simulink library "inp"  (R2021b)
settings: Solver=VariableStepAuto  StartTime=0.0  StopTime=10.0  RelTol=1e-3
undefined symbols (not defined in the file): C_TASK_5MS_S, FALSE, KINP_AcoreReadyToSlp_flg_ovrdflg, KINP_AcoreReadyToSlp_flg_ovrdval, KINP_AllowMovThd_OTA_enum_ovrdflg, KINP_AllowMovThd_OTA_enum_ovrdval, KINP_APSAngleTarget_Deg_ovrdflg, KINP_APSAngleTarget_Deg_ovrdval, KINP_APSDecReq_mps2_ovrdflg, KINP_APSDecReq_mps2_ovrdval, KINP_APSDecReqA_flg_ovrdflg, KINP_APSDecReqA_flg_ovrdval, KINP_APSDFLL_cm_ovrdflg, KINP_APSDFLL_cm_ovrdval, KINP_APSDFLR_cm_ovrdflg, KINP_APSDFLR_cm_ovrdval, KINP_APSDRLL_cm_ovrdflg, KINP_APSDRLL_cm_ovrdval, KINP_APSDRLR_cm_ovrdflg, KINP_APSDRLR_cm_ovrdval, KINP_APSExitCondition_enum_ovrdflg, KINP_APSExitCondition_enum_ovrdval, KINP_APSHWVer_enum_ovrdflg, KINP_APSHWVer_enum_ovrdval, KINP_APSProgressPCT_pct_ovrdflg, KINP_APSProgressPCT_pct_ovrdval, KINP_APSPwrReq_enum_ovrdflg, KINP_APSPwrReq_enum_ovrdval, KINP_APSReq_enum_ovrdflg, KINP_APSReq_enum_ovrdval, KINP_APSRQDisplay_enum_ovrdflg, KINP_APSRQDisplay_enum_ovrdval, KINP_APSRqEPASCtrl_flg_ovrdflg, KINP_APSRqEPASCtrl_flg_ovrdval, KINP_APSShiftPosnReq_enum_ovrdval, KINP_APSShiftPosnReq_enum_ovrflg, KINP_APSSpeedCMD_kph_ovrdval, KINP_APSSpeedCMD_kph_ovrflg, KINP_APSStaSystem_enum_ovrdflg, KINP_APSStaSystem_enum_ovrdval, KINP_APSSWVer_enum_ovrdflg, KINP_APSSWVer_enum_ovrdval, KINP_APSVMCReqA_flg_ovrdval, KINP_APSVMCReqA_flg_ovrflg, KINP_APSVRqEPASCtrl_flg_ovrdflg, KINP_APSVRqEPASCtrl_flg_ovrdval, KINP_AuxBattVolmV_mV_ovrdflg, KINP_AuxBattVolmV_mV_ovrdval, KINP_CAASSta_enum_ovrdflg, KINP_CAASSta_enum_ovrdval, KINP_CAASVMCReqA_flg_ovrdval, KINP_CAASVMCReqA_flg_ovrflg, KINP_CAN1BusOff_flg_ovrdflg, KINP_CAN1BusOff_flg_ovrdval, KINP_CAN2BusOff_flg_ovrdflg, KINP_CAN2BusOff_flg_ovrdval, KINP_CAN3BusOff_flg_ovrdflg, KINP_CAN3BusOff_flg_ovrdval, KINP_CAN4BusOff_flg_ovrdflg, KINP_CAN4BusOff_flg_ovrdval ... (+152)
libraries: FVT_lib x1035, hcu_lib x1
(part 27 of 33)

== system inp/INP/CAN4/SignalCheck/ZONE_FR1 ==
  BHAL_outputs : Inport
  inp_CanValid_bus : Inport  Port=2
  ChargeInletLockSta : FVT_lib/inp/can_signal_template  SystemSampleTime=-1  VariantActivationTime=update diagram  Latency=0  AutoFrameSizeCalculation=off
      link override defval: Value=KINP_ChargeInletLockSta_flg_defval
      link override ovrdflg: Value=KINP_ChargeInletLockSta_flg_ovrdflg
      link override ovrdval: Value=KINP_ChargeInletLockSta_flg_ovrdval
  CompProEN : FVT_lib/inp/can_signal_template  SystemSampleTime=-1  VariantActivationTime=update diagram  Latency=0  AutoFrameSizeCalculation=off
      link override defval: Value=KINP_CompProEN_flg_defval
      link override ovrdflg: Value=KINP_CompProEN_flg_ovrdflg
      link override ovrdval: Value=KINP_CompProEN_flg_ovrdval
  FLTurnLPErr : FVT_lib/inp/can_signal_template  SystemSampleTime=-1  VariantActivationTime=update diagram  Latency=0  AutoFrameSizeCalculation=off
      link override defval: Value=KINP_FLTurnLPErr_flg_defval
      link override ovrdflg: Value=KINP_FLTurnLPErr_flg_ovrdflg
      link override ovrdval: Value=KINP_FLTurnLPErr_flg_ovrdval
  FLTurnLampC : FVT_lib/inp/can_signal_template  SystemSampleTime=-1  VariantActivationTime=update diagram  Latency=0  AutoFrameSizeCalculation=off
      link override defval: Value=KINP_FLTurnLampC_mA_defval
      link override ovrdflg: Value=KINP_FLTurnLampC_mA_ovrdflg
      link override ovrdval: Value=KINP_FLTurnLampC_mA_ovrdval
  FLTurnLightWarning : FVT_lib/inp/can_signal_template  SystemSampleTime=-1  VariantActivationTime=update diagram  Latency=0  AutoFrameSizeCalculation=off
      link override defval: Value=KINP_FLTurnLightWarning_flg_defval
      link override ovrdflg: Value=KINP_FLTurnLightWarning_flg_ovrdflg
      link override ovrdval: Value=KINP_FLTurnLightWarning_flg_ovrdval
  FRTurnLPErr : FVT_lib/inp/can_signal_template  SystemSampleTime=-1  VariantActivationTime=update diagram  Latency=0  AutoFrameSizeCalculation=off
      link override defval: Value=KINP_FRTurnLPErr_flg_defval
      link override ovrdflg: Value=KINP_FRTurnLPErr_flg_ovrdflg
      link override ovrdval: Value=KINP_FRTurnLPErr_flg_ovrdval
  FRTurnLampC : FVT_lib/inp/can_signal_template  SystemSampleTime=-1  VariantActivationTime=update diagram  Latency=0  AutoFrameSizeCalculation=off
      link override defval: Value=KINP_FRTurnLampC_mA_defval
      link override ovrdflg: Value=KINP_FRTurnLampC_mA_ovrdflg
      link override ovrdval: Value=KINP_FRTurnLampC_mA_ovrdval
  FRTurnLightWarning : FVT_lib/inp/can_signal_template  SystemSampleTime=-1  VariantActivationTime=update diagram  Latency=0  AutoFrameSizeCalculation=off
      link override defval: Value=KINP_FRTurnLightWarning_flg_defval
      link override ovrdflg: Value=KINP_FRTurnLightWarning_flg_ovrdflg
      link override ovrdval: Value=KINP_FRTurnLightWarning_flg_ovrdval
  FWiperAS : FVT_lib/inp/can_signal_template  SystemSampleTime=-1  VariantActivationTime=update diagram  Latency=0  AutoFrameSizeCalculation=off
      link override defval: Value=KINP_FWiperAS_flg_defval
      link override ovrdflg: Value=KINP_FWiperAS_flg_ovrdflg
      link override ovrdval: Value=KINP_FWiperAS_flg_ovrdval
  FWiperProtection : FVT_lib/inp/can_signal_template  SystemSampleTime=-1  VariantActivationTime=update diagram  Latency=0  AutoFrameSizeCalculation=off
      link override defval: Value=KINP_FWiperProtection_flg_defval
      link override ovrdflg: Value=KINP_FWiperProtection_flg_ovrdflg
      link override ovrdval: Value=KINP_FWiperProtection_flg_ovrdval
  LADBHibeamIndication : FVT_lib/inp/can_signal_template  SystemSampleTime=-1  VariantActivationTime=update diagram  Latency=0  AutoFrameSizeCalculation=off
      link override defval: Value=KINP_LADBHibeamIndication_flg_defval
      link override ovrdflg: Value=KINP_LADBHibeamIndication_flg_ovrdflg
      link override ovrdval: Value=KINP_LADBHibeamIndication_flg_ovrdval
  LADBOperationStatus : FVT_lib/inp/can_signal_template  SystemSampleTime=-1  VariantActivationTime=update diagram  Latency=0  AutoFrameSizeCalculation=off
      link override defval: Value=KINP_LADBOperationStatus_flg_defval
      link override ovrdflg: Value=KINP_LADBOperationStatus_flg_ovrdflg
      link override ovrdval: Value=KINP_LADBOperationStatus_flg_ovrdval
  LADBWarning : FVT_lib/inp/can_signal_template  SystemSampleTime=-1  VariantActivationTime=update diagram  Latency=0  AutoFrameSizeCalculation=off
      link override defval: Value=KINP_LADBWarning_flg_defval
      link override ovrdflg: Value=KINP_LADBWarning_flg_ovrdflg
      link override ovrdval: Value=KINP_LADBWarning_flg_ovrdval
  LAHBWarning : FVT_lib/inp/can_signal_template  SystemSampleTime=-1  VariantActivationTime=update diagram  Latency=0  AutoFrameSizeCalculation=off
      link override defval: Value=KINP_LAHBWarning_flg_defval
      link override ovrdflg: Value=KINP_LAHBWarning_flg_ovrdflg
      link override ovrdval: Value=KINP_LAHBWarning_flg_ovrdval
  LDRLWarning : FVT_lib/inp/can_signal_template  SystemSampleTime=-1  VariantActivationTime=update diagram  Latency=0  AutoFrameSizeCalculation=off
      link override defval: Value=KINP_LDRLWarning_flg_defval
      link override ovrdflg: Value=KINP_LDRLWarning_flg_ovrdflg
      link override ovrdval: Value=KINP_LDRLWarning_flg_ovrdval
  LLBWarning : FVT_lib/inp/can_signal_template  SystemSampleTime=-1  VariantActivationTime=update diagram  Latency=0  AutoFrameSizeCalculation=off
      link override defval: Value=KINP_LLBWarning_flg_defval
      link override ovrdflg: Value=KINP_LLBWarning_flg_ovrdflg
      link override ovrdval: Value=KINP_LLBWarning_flg_ovrdval
  LpositionLampWarning : FVT_lib/inp/can_signal_template  SystemSampleTime=-1  VariantActivationTime=update diagram  Latency=0  AutoFrameSizeCalculation=off
      link override defval: Value=KINP_LpositionLampWarning_flg_defval
      link override ovrdflg: Value=KINP_LpositionLampWarning_flg_ovrdflg
      link override ovrdval: Value=KINP_LpositionLampWarning_flg_ovrdval
  RADBHibeamIndication : FVT_lib/inp/can_signal_template  SystemSampleTime=-1  VariantActivationTime=update diagram  Latency=0  AutoFrameSizeCalculation=off
      link override defval: Value=KINP_RADBHibeamIndication_flg_defval
      link override ovrdflg: Value=KINP_RADBHibeamIndication_flg_ovrdflg
      link override ovrdval: Value=KINP_RADBHibeamIndication_flg_ovrdval
  RADBOperationStatus : FVT_lib/inp/can_signal_template  SystemSampleTime=-1  VariantActivationTime=update diagram  Latency=0  AutoFrameSizeCalculation=off
      link override defval: Value=KINP_RADBOperationStatus_flg_defval
      link override ovrdflg: Value=KINP_RADBOperationStatus_flg_ovrdflg
      link override ovrdval: Value=KINP_RADBOperationStatus_flg_ovrdval
  RADBWarning : FVT_lib/inp/can_signal_template  SystemSampleTime=-1  VariantActivationTime=update diagram  Latency=0  AutoFrameSizeCalculation=off
      link override defval: Value=KINP_RADBWarning_flg_defval
      link override ovrdflg: Value=KINP_RADBWarning_flg_ovrdflg
      link override ovrdval: Value=KINP_RADBWarning_flg_ovrdval
  RAHBWarning : FVT_lib/inp/can_signal_template  SystemSampleTime=-1  VariantActivationTime=update diagram  Latency=0  AutoFrameSizeCalculation=off
      link override defval: Value=KINP_RAHBWarning_flg_defval
      link override ovrdflg: Value=KINP_RAHBWarning_flg_ovrdflg
      link override ovrdval: Value=KINP_RAHBWarning_flg_ovrdval
  RDRLWarning : FVT_lib/inp/can_signal_template  SystemSampleTime=-1  VariantActivationTime=update diagram  Latency=0  AutoFrameSizeCalculation=off
      link override defval: Value=KINP_RDRLWarning_flg_defval
      link override ovrdflg: Value=KINP_RDRLWarning_flg_ovrdflg
      link override ovrdval: Value=KINP_RDRLWarning_flg_ovrdval
  RLBWarning : FVT_lib/inp/can_signal_template  SystemSampleTime=-1  VariantActivationTime=update diagram  Latency=0  AutoFrameSizeCalculation=off
      link override defval: Value=KINP_RLBWarning_flg_defval
      link override ovrdflg: Value=KINP_RLBWarning_flg_ovrdflg
      link override ovrdval: Value=KINP_RLBWarning_flg_ovrdval
  RpositionLampWarning : FVT_lib/inp/can_signal_template  SystemSampleTime=-1  VariantActivationTime=update diagram  Latency=0  AutoFrameSizeCalculation=off
      link override defval: Value=KINP_RpositionLampWarning_flg_defval
      link override ovrdflg: Value=KINP_RpositionLampWarning_flg_ovrdflg
      link override ovrdval: Value=KINP_RpositionLampWarning_flg_ovrdval
  Terminator_{1..33} (33 alike) : Terminator
  TrailerCheck : FVT_lib/inp/can_signal_template  SystemSampleTime=-1  VariantActivationTime=update diagram  Latency=0  AutoFrameSizeCalculation=off
      link override defval: Value=KINP_TrailerCheck_flg_defval
      link override ovrdflg: Value=KINP_TrailerCheck_flg_ovrdflg
      link override ovrdval: Value=KINP_TrailerCheck_flg_ovrdval
  TrailerModeSta : FVT_lib/inp/can_signal_template  SystemSampleTime=-1  VariantActivationTime=update diagram  Latency=0  AutoFrameSizeCalculation=off
      link override defval: Value=KINP_TrailerModeSta_enum_defval
      link override ovrdflg: Value=KINP_TrailerModeSta_enum_ovrdflg
      link override ovrdval: Value=KINP_TrailerModeSta_enum_ovrdval
  True_VHAL_ChargeInletLockSta_flg : Constant  Value=TRUE  OutDataTypeStr=boolean
  True_VHAL_CompProEN_flg : Constant  Value=TRUE  OutDataTypeStr=boolean
  True_VHAL_FLTurnLPErr_flg : Constant  Value=TRUE  OutDataTypeStr=boolean
  True_VHAL_FLTurnLampC_mA : Constant  Value=TRUE  OutDataTypeStr=boolean
  True_VHAL_FLTurnLightWarning_flg : Constant  Value=TRUE  OutDataTypeStr=boolean
  True_VHAL_FRTurnLPErr_flg : Constant  Value=TRUE  OutDataTypeStr=boolean
  True_VHAL_FRTurnLampC_mA : Constant  Value=TRUE  OutDataTypeStr=boolean
  True_VHAL_FRTurnLightWarning_flg : Constant  Value=TRUE  OutDataTypeStr=boolean
  True_VHAL_FWiperAS_flg : Constant  Value=TRUE  OutDataTypeStr=boolean
  True_VHAL_FWiperProtection_flg : Constant  Value=TRUE  OutDataTypeStr=boolean
  True_VHAL_LADBHibeamIndication_flg : Constant  Value=TRUE  OutDataTypeStr=boolean
  True_VHAL_LADBOperationStatus_flg : Constant  Value=TRUE  OutDataTypeStr=boolean
  True_VHAL_LADBWarning_flg : Constant  Value=TRUE  OutDataTypeStr=boolean
  True_VHAL_LAHBWarning_flg : Constant  Value=TRUE  OutDataTypeStr=boolean
  True_VHAL_LDRLWarning_flg : Constant  Value=TRUE  OutDataTypeStr=boolean
  True_VHAL_LLBWarning_flg : Constant  Value=TRUE  OutDataTypeStr=boolean
  True_VHAL_LpositionLampWarning_flg : Constant  Value=TRUE  OutDataTypeStr=boolean
  True_VHAL_RADBHibeamIndication_flg : Constant  Value=TRUE  OutDataTypeStr=boolean
  True_VHAL_RADBOperationStatus_flg : Constant  Value=TRUE  OutDataTypeStr=boolean
  True_VHAL_RADBWarning_flg : Constant  Value=TRUE  OutDataTypeStr=boolean
  True_VHAL_RAHBWarning_flg : Constant  Value=TRUE  OutDataTypeStr=boolean
  True_VHAL_RDRLWarning_flg : Constant  Value=TRUE  OutDataTypeStr=boolean
  True_VHAL_RLBWarning_flg : Constant  Value=TRUE  OutDataTypeStr=boolean
  True_VHAL_RpositionLampWarning_flg : Constant  Value=TRUE  OutDataTypeStr=boolean
  True_VHAL_TrailerCheck_flg : Constant  Value=TRUE  OutDataTypeStr=boolean
  True_VHAL_TrailerModeSta_enum : Constant  Value=TRUE  OutDataTypeStr=boolean
  True_VHAL_ZFRBCMChargerDoorSWSta_flg : Constant  Value=TRUE  OutDataTypeStr=boolean
  True_VHAL_ZFRBCMHRLTurnLPNormalSta_flg : Constant  Value=TRUE  OutDataTypeStr=boolean
  True_VHAL_ZFRBCMHRRTurnLPHNormalSta_flg : Constant  Value=TRUE  OutDataTypeStr=boolean
  True_VHAL_ZFRTHCMCLEVentActYSta_pct : Constant  Value=TRUE  OutDataTypeStr=boolean
  True_VHAL_ZFRTHCMCREVentActYSta_pct : Constant  Value=TRUE  OutDataTypeStr=boolean
  True_VHAL_ZFRTHCMDrEVentActYSta_pct : Constant  Value=TRUE  OutDataTypeStr=boolean
  True_VHAL_ZFRTHCMPsEVentActYSta_pct : Constant  Value=TRUE  OutDataTypeStr=boolean
  ZFRBCMChargerDoorSWSta : FVT_lib/inp/can_signal_template  SystemSampleTime=-1  VariantActivationTime=update diagram  Latency=0  AutoFrameSizeCalculation=off
      link override defval: Value=KINP_ZFRBCMChargerDoorSWSta_flg_defval
      link override ovrdflg: Value=KINP_ZFRBCMChargerDoorSWSta_flg_ovrdflg
      link override ovrdval: Value=KINP_ZFRBCMChargerDoorSWSta_flg_ovrdval
  ZFRBCMHRLTurnLPNormalSta : FVT_lib/inp/can_signal_template  SystemSampleTime=-1  VariantActivationTime=update diagram  Latency=0  AutoFrameSizeCalculation=off
      link override defval: Value=KINP_ZFRBCMHRLTurnLPNormalSta_flg_defval
      link override ovrdflg: Value=KINP_ZFRBCMHRLTurnLPNormalSta_flg_ovrdflg
      link override ovrdval: Value=KINP_ZFRBCMHRLTurnLPNormalSta_flg_ovrdval
  ZFRBCMHRRTurnLPHNormalSta : FVT_lib/inp/can_signal_template  SystemSampleTime=-1  VariantActivationTime=update diagram  Latency=0  AutoFrameSizeCalculation=off
      link override defval: Value=KINP_ZFRBCMHRRTurnLPHNormalSta_flg_defval
      link override ovrdflg: Value=KINP_ZFRBCMHRRTurnLPHNormalSta_flg_ovrdflg
      link override ovrdval: Value=KINP_ZFRBCMHRRTurnLPHNormalSta_flg_ovrdval
  ZFRTHCMCLEVentActYSta : FVT_lib/inp/can_signal_template  SystemSampleTime=-1  VariantActivationTime=update diagram  Latency=0  AutoFrameSizeCalculation=off
      link override defval: Value=KINP_ZFRTHCMCLEVentActYSta_pct_defval
      link override ovrdflg: Value=KINP_ZFRTHCMCLEVentActYSta_pct_ovrdflg
      link override ovrdval: Value=KINP_ZFRTHCMCLEVentActYSta_pct_ovrdval
  ZFRTHCMCREVentActYSta : FVT_lib/inp/can_signal_template  SystemSampleTime=-1  VariantActivationTime=update diagram  Latency=0  AutoFrameSizeCalculation=off
      link override defval: Value=KINP_ZFRTHCMCREVentActYSta_pct_defval
      link override ovrdflg: Value=KINP_ZFRTHCMCREVentActYSta_pct_ovrdflg
      link override ovrdval: Value=KINP_ZFRTHCMCREVentActYSta_pct_ovrdval
  ZFRTHCMDrEVentActYSta : FVT_lib/inp/can_signal_template  SystemSampleTime=-1  VariantActivationTime=update diagram  Latency=0  AutoFrameSizeCalculation=off
      link override defval: Value=KINP_ZFRTHCMDrEVentActYSta_pct_defval
      link override ovrdflg: Value=KINP_ZFRTHCMDrEVentActYSta_pct_ovrdflg
      link override ovrdval: Value=KINP_ZFRTHCMDrEVentActYSta_pct_ovrdval
  ZFRTHCMPsEVentActYSta : FVT_lib/inp/can_signal_template  SystemSampleTime=-1  VariantActivationTime=update diagram  Latency=0  AutoFrameSizeCalculation=off
      link override defval: Value=KINP_ZFRTHCMPsEVentActYSta_pct_defval
      link override ovrdflg: Value=KINP_ZFRTHCMPsEVentActYSta_pct_ovrdflg
      link override ovrdval: Value=KINP_ZFRTHCMPsEVentActYSta_pct_ovrdval
  slr1_{1..33} (33 alike) : BusSelector  OutputSignals=VINP_CANMsgValidZONEFR1_flg
  slr_VHAL_ChargeInletLockSta_flg : BusSelector  OutputSignals=VHAL_ChargeInletLockSta_flg
  slr_VHAL_CompProEN_flg : BusSelector  OutputSignals=VHAL_CompProEN_flg
  slr_VHAL_FLTurnLPErr_flg : BusSelector  OutputSignals=VHAL_FLTurnLPErr_flg
  slr_VHAL_FLTurnLampC_mA : BusSelector  OutputSignals=VHAL_FLTurnLampC_mA
  slr_VHAL_FLTurnLightWarning_flg : BusSelector  OutputSignals=VHAL_FLTurnLightWarning_flg
  slr_VHAL_FRTurnLPErr_flg : BusSelector  OutputSignals=VHAL_FRTurnLPErr_flg
  slr_VHAL_FRTurnLampC_mA : BusSelector  OutputSignals=VHAL_FRTurnLampC_mA
  slr_VHAL_FRTurnLightWarning_flg : BusSelector  OutputSignals=VHAL_FRTurnLightWarning_flg
  slr_VHAL_FWiperAS_flg : BusSelector  OutputSignals=VHAL_FWiperAS_flg
  slr_VHAL_FWiperProtection_flg : BusSelector  OutputSignals=VHAL_FWiperProtection_flg
  slr_VHAL_LADBHibeamIndication_flg : BusSelector  OutputSignals=VHAL_LADBHibeamIndication_flg
  slr_VHAL_LADBOperationStatus_flg : BusSelector  OutputSignals=VHAL_LADBOperationStatus_flg
  slr_VHAL_LADBWarning_flg : BusSelector  OutputSignals=VHAL_LADBWarning_flg
  slr_VHAL_LAHBWarning_flg : BusSelector  OutputSignals=VHAL_LAHBWarning_flg
  slr_VHAL_LDRLWarning_flg : BusSelector  OutputSignals=VHAL_LDRLWarning_flg
  slr_VHAL_LLBWarning_flg : BusSelector  OutputSignals=VHAL_LLBWarning_flg
  slr_VHAL_LpositionLampWarning_flg : BusSelector  OutputSignals=VHAL_LpositionLampWarning_flg
  slr_VHAL_RADBHibeamIndication_flg : BusSelector  OutputSignals=VHAL_RADBHibeamIndication_flg
  slr_VHAL_RADBOperationStatus_flg : BusSelector  OutputSignals=VHAL_RADBOperationStatus_flg
  slr_VHAL_RADBWarning_flg : BusSelector  OutputSignals=VHAL_RADBWarning_flg
  slr_VHAL_RAHBWarning_flg : BusSelector  OutputSignals=VHAL_RAHBWarning_flg
  slr_VHAL_RDRLWarning_flg : BusSelector  OutputSignals=VHAL_RDRLWarning_flg
  slr_VHAL_RLBWarning_flg : BusSelector  OutputSignals=VHAL_RLBWarning_flg
  slr_VHAL_RpositionLampWarning_flg : BusSelector  OutputSignals=VHAL_RpositionLampWarning_flg
  slr_VHAL_TrailerCheck_flg : BusSelector  OutputSignals=VHAL_TrailerCheck_flg
  slr_VHAL_TrailerModeSta_enum : BusSelector  OutputSignals=VHAL_TrailerModeSta_enum
  slr_VHAL_ZFRBCMChargerDoorSWSta_flg : BusSelector  OutputSignals=VHAL_ZFRBCMChargerDoorSWSta_flg
  slr_VHAL_ZFRBCMHRLTurnLPNormalSta_flg : BusSelector  OutputSignals=VHAL_ZFRBCMHRLTurnLPNormalSta_flg
  slr_VHAL_ZFRBCMHRRTurnLPHNormalSta_flg : BusSelector  OutputSignals=VHAL_ZFRBCMHRRTurnLPHNormalSta_flg
  slr_VHAL_ZFRTHCMCLEVentActYSta_pct : BusSelector  OutputSignals=VHAL_ZFRTHCMCLEVentActYSta_pct
  slr_VHAL_ZFRTHCMCREVentActYSta_pct : BusSelector  OutputSignals=VHAL_ZFRTHCMCREVentActYSta_pct
  slr_VHAL_ZFRTHCMDrEVentActYSta_pct : BusSelector  OutputSignals=VHAL_ZFRTHCMDrEVentActYSta_pct
  slr_VHAL_ZFRTHCMPsEVentActYSta_pct : BusSelector  OutputSignals=VHAL_ZFRTHCMPsEVentActYSta_pct
  VINP_ChargeInletLockSta_flg : Outport
  VINP_CompProEN_flg : Outport  Port=2
  VINP_FLTurnLPErr_flg : Outport  Port=3
  VINP_FLTurnLampC_mA : Outport  Port=4
  VINP_FLTurnLightWarning_flg : Outport  Port=5
  VINP_FRTurnLPErr_flg : Outport  Port=6
  VINP_FRTurnLampC_mA : Outport  Port=7
  VINP_FRTurnLightWarning_flg : Outport  Port=8
  VINP_FWiperAS_flg : Outport  Port=9
  VINP_FWiperProtection_flg : Outport  Port=10
  VINP_LADBHibeamIndication_flg : Outport  Port=11
  VINP_LADBOperationStatus_flg : Outport  Port=12
  VINP_LADBWarning_flg : Outport  Port=13
  VINP_LAHBWarning_flg : Outport  Port=14
  VINP_LDRLWarning_flg : Outport  Port=15
  VINP_LLBWarning_flg : Outport  Port=16
  VINP_LpositionLampWarning_flg : Outport  Port=17
  VINP_RADBHibeamIndication_flg : Outport  Port=18
  VINP_RADBOperationStatus_flg : Outport  Port=19
  VINP_RADBWarning_flg : Outport  Port=20
  VINP_RAHBWarning_flg : Outport  Port=21
  VINP_RDRLWarning_flg : Outport  Port=22
  VINP_RLBWarning_flg : Outport  Port=23
  VINP_RpositionLampWarning_flg : Outport  Port=24
  VINP_TrailerCheck_flg : Outport  Port=25
  VINP_TrailerModeSta_enum : Outport  Port=26
  VINP_ZFRBCMChargerDoorSWSta_flg : Outport  Port=27
  VINP_ZFRBCMHRLTurnLPNormalSta_flg : Outport  Port=28
  VINP_ZFRBCMHRRTurnLPHNormalSta_flg : Outport  Port=29
  VINP_ZFRTHCMCLEVentActYSta_pct : Outport  Port=30
  VINP_ZFRTHCMCREVentActYSta_pct : Outport  Port=31
  VINP_ZFRTHCMDrEVentActYSta_pct : Outport  Port=32
  VINP_ZFRTHCMPsEVentActYSta_pct : Outport  Port=33
  wires:
  BHAL_outputs/1 -> [BHAL_outputs]
  inp_CanValid_bus/1 -> [inp_CanValid_bus]
  [BHAL_outputs] -> slr_VHAL_ChargeInletLockSta_flg/1
  slr_VHAL_ChargeInletLockSta_flg/1 -> ChargeInletLockSta/1  "<VHAL_ChargeInletLockSta_flg>"
  True_VHAL_ChargeInletLockSta_flg/1 -> ChargeInletLockSta/2
  [inp_CanValid_bus] -> slr1_1/1
  slr1_1/1 -> ChargeInletLockSta/3  "<VINP_CANMsgValidZONEFR1_flg>"
  ChargeInletLockSta/1 -> VINP_ChargeInletLockSta_flg/1  "VINP_ChargeInletLockSta_flg"
  ChargeInletLockSta/2 -> Terminator_1/1
  [BHAL_outputs] -> slr_VHAL_CompProEN_flg/1
  slr_VHAL_CompProEN_flg/1 -> CompProEN/1  "<VHAL_CompProEN_flg>"
  True_VHAL_CompProEN_flg/1 -> CompProEN/2
  [inp_CanValid_bus] -> slr1_2/1
  slr1_2/1 -> CompProEN/3  "<VINP_CANMsgValidZONEFR1_flg>"
  CompProEN/1 -> VINP_CompProEN_flg/1  "VINP_CompProEN_flg"
  CompProEN/2 -> Terminator_2/1
  [BHAL_outputs] -> slr_VHAL_FLTurnLPErr_flg/1
  slr_VHAL_FLTurnLPErr_flg/1 -> FLTurnLPErr/1  "<VHAL_FLTurnLPErr_flg>"
  True_VHAL_FLTurnLPErr_flg/1 -> FLTurnLPErr/2
  [inp_CanValid_bus] -> slr1_3/1
  slr1_3/1 -> FLTurnLPErr/3  "<VINP_CANMsgValidZONEFR1_flg>"
  FLTurnLPErr/1 -> VINP_FLTurnLPErr_flg/1  "VINP_FLTurnLPErr_flg"
  FLTurnLPErr/2 -> Terminator_3/1
  [BHAL_outputs] -> slr_VHAL_FLTurnLampC_mA/1
  slr_VHAL_FLTurnLampC_mA/1 -> FLTurnLampC/1  "<VHAL_FLTurnLampC_mA>"
  True_VHAL_FLTurnLampC_mA/1 -> FLTurnLampC/2
  [inp_CanValid_bus] -> slr1_4/1
  slr1_4/1 -> FLTurnLampC/3  "<VINP_CANMsgValidZONEFR1_flg>"
  FLTurnLampC/1 -> VINP_FLTurnLampC_mA/1  "VINP_FLTurnLampC_mA"
  FLTurnLampC/2 -> Terminator_4/1
  [BHAL_outputs] -> slr_VHAL_FLTurnLightWarning_flg/1
  slr_VHAL_FLTurnLightWarning_flg/1 -> FLTurnLightWarning/1  "<VHAL_FLTurnLightWarning_flg>"
  True_VHAL_FLTurnLightWarning_flg/1 -> FLTurnLightWarning/2
  [inp_CanValid_bus] -> slr1_5/1
  slr1_5/1 -> FLTurnLightWarning/3  "<VINP_CANMsgValidZONEFR1_flg>"
  FLTurnLightWarning/1 -> VINP_FLTurnLightWarning_flg/1  "VINP_FLTurnLightWarning_flg"
  FLTurnLightWarning/2 -> Terminator_5/1
  [BHAL_outputs] -> slr_VHAL_FRTurnLPErr_flg/1
  slr_VHAL_FRTurnLPErr_flg/1 -> FRTurnLPErr/1  "<VHAL_FRTurnLPErr_flg>"
  True_VHAL_FRTurnLPErr_flg/1 -> FRTurnLPErr/2
  [inp_CanValid_bus] -> slr1_6/1
  slr1_6/1 -> FRTurnLPErr/3  "<VINP_CANMsgValidZONEFR1_flg>"
  FRTurnLPErr/1 -> VINP_FRTurnLPErr_flg/1  "VINP_FRTurnLPErr_flg"
  FRTurnLPErr/2 -> Terminator_6/1
  [BHAL_outputs] -> slr_VHAL_FRTurnLampC_mA/1
  slr_VHAL_FRTurnLampC_mA/1 -> FRTurnLampC/1  "<VHAL_FRTurnLampC_mA>"
  True_VHAL_FRTurnLampC_mA/1 -> FRTurnLampC/2
  [inp_CanValid_bus] -> slr1_7/1
  slr1_7/1 -> FRTurnLampC/3  "<VINP_CANMsgValidZONEFR1_flg>"
  FRTurnLampC/1 -> VINP_FRTurnLampC_mA/1  "VINP_FRTurnLampC_mA"
  FRTurnLampC/2 -> Terminator_7/1
  [BHAL_outputs] -> slr_VHAL_FRTurnLightWarning_flg/1
  slr_VHAL_FRTurnLightWarning_flg/1 -> FRTurnLightWarning/1  "<VHAL_FRTurnLightWarning_flg>"
  True_VHAL_FRTurnLightWarning_flg/1 -> FRTurnLightWarning/2
  [inp_CanValid_bus] -> slr1_8/1
  slr1_8/1 -> FRTurnLightWarning/3  "<VINP_CANMsgValidZONEFR1_flg>"
  FRTurnLightWarning/1 -> VINP_FRTurnLightWarning_flg/1  "VINP_FRTurnLightWarning_flg"
  FRTurnLightWarning/2 -> Terminator_8/1
  [BHAL_outputs] -> slr_VHAL_FWiperAS_flg/1
  slr_VHAL_FWiperAS_flg/1 -> FWiperAS/1  "<VHAL_FWiperAS_flg>"
  True_VHAL_FWiperAS_flg/1 -> FWiperAS/2
  [inp_CanValid_bus] -> slr1_9/1
  slr1_9/1 -> FWiperAS/3  "<VINP_CANMsgValidZONEFR1_flg>"
  FWiperAS/1 -> VINP_FWiperAS_flg/1  "VINP_FWiperAS_flg"
  FWiperAS/2 -> Terminator_9/1
  [BHAL_outputs] -> slr_VHAL_FWiperProtection_flg/1
  slr_VHAL_FWiperProtection_flg/1 -> FWiperProtection/1  "<VHAL_FWiperProtection_flg>"
  True_VHAL_FWiperProtection_flg/1 -> FWiperProtection/2
  [inp_CanValid_bus] -> slr1_10/1
  slr1_10/1 -> FWiperProtection/3  "<VINP_CANMsgValidZONEFR1_flg>"
  FWiperProtection/1 -> VINP_FWiperProtection_flg/1  "VINP_FWiperProtection_flg"
  FWiperProtection/2 -> Terminator_10/1
  [BHAL_outputs] -> slr_VHAL_LADBHibeamIndication_flg/1
  slr_VHAL_LADBHibeamIndication_flg/1 -> LADBHibeamIndication/1  "<VHAL_LADBHibeamIndication_flg>"
  True_VHAL_LADBHibeamIndication_flg/1 -> LADBHibeamIndication/2
  [inp_CanValid_bus] -> slr1_11/1
  slr1_11/1 -> LADBHibeamIndication/3  "<VINP_CANMsgValidZONEFR1_flg>"
  LADBHibeamIndication/1 -> VINP_LADBHibeamIndication_flg/1  "VINP_LADBHibeamIndication_flg"
  LADBHibeamIndication/2 -> Terminator_11/1
  [BHAL_outputs] -> slr_VHAL_LADBOperationStatus_flg/1
  slr_VHAL_LADBOperationStatus_flg/1 -> LADBOperationStatus/1  "<VHAL_LADBOperationStatus_flg>"
  True_VHAL_LADBOperationStatus_flg/1 -> LADBOperationStatus/2
  [inp_CanValid_bus] -> slr1_12/1
  slr1_12/1 -> LADBOperationStatus/3  "<VINP_CANMsgValidZONEFR1_flg>"
  LADBOperationStatus/1 -> VINP_LADBOperationStatus_flg/1  "VINP_LADBOperationStatus_flg"
  LADBOperationStatus/2 -> Terminator_12/1
  [BHAL_outputs] -> slr_VHAL_LADBWarning_flg/1
  slr_VHAL_LADBWarning_flg/1 -> LADBWarning/1  "<VHAL_LADBWarning_flg>"
  True_VHAL_LADBWarning_flg/1 -> LADBWarning/2
  [inp_CanValid_bus] -> slr1_13/1
  slr1_13/1 -> LADBWarning/3  "<VINP_CANMsgValidZONEFR1_flg>"
  LADBWarning/1 -> VINP_LADBWarning_flg/1  "VINP_LADBWarning_flg"
  LADBWarning/2 -> Terminator_13/1
  [BHAL_outputs] -> slr_VHAL_LAHBWarning_flg/1
  slr_VHAL_LAHBWarning_flg/1 -> LAHBWarning/1  "<VHAL_LAHBWarning_flg>"
  True_VHAL_LAHBWarning_flg/1 -> LAHBWarning/2
  [inp_CanValid_bus] -> slr1_14/1
  slr1_14/1 -> LAHBWarning/3  "<VINP_CANMsgValidZONEFR1_flg>"
  LAHBWarning/1 -> VINP_LAHBWarning_flg/1  "VINP_LAHBWarning_flg"
  LAHBWarning/2 -> Terminator_14/1
  [BHAL_outputs] -> slr_VHAL_LDRLWarning_flg/1
  slr_VHAL_LDRLWarning_flg/1 -> LDRLWarning/1  "<VHAL_LDRLWarning_flg>"
  True_VHAL_LDRLWarning_flg/1 -> LDRLWarning/2
  [inp_CanValid_bus] -> slr1_15/1
  slr1_15/1 -> LDRLWarning/3  "<VINP_CANMsgValidZONEFR1_flg>"
  LDRLWarning/1 -> VINP_LDRLWarning_flg/1  "VINP_LDRLWarning_flg"
  LDRLWarning/2 -> Terminator_15/1
  [BHAL_outputs] -> slr_VHAL_LLBWarning_flg/1
  slr_VHAL_LLBWarning_flg/1 -> LLBWarning/1  "<VHAL_LLBWarning_flg>"
  True_VHAL_LLBWarning_flg/1 -> LLBWarning/2
  [inp_CanValid_bus] -> slr1_16/1
  slr1_16/1 -> LLBWarning/3  "<VINP_CANMsgValidZONEFR1_flg>"
  LLBWarning/1 -> VINP_LLBWarning_flg/1  "VINP_LLBWarning_flg"
  LLBWarning/2 -> Terminator_16/1
  [BHAL_outputs] -> slr_VHAL_LpositionLampWarning_flg/1
  slr_VHAL_LpositionLampWarning_flg/1 -> LpositionLampWarning/1  "<VHAL_LpositionLampWarning_flg>"
  True_VHAL_LpositionLampWarning_flg/1 -> LpositionLampWarning/2
  [inp_CanValid_bus] -> slr1_17/1
  slr1_17/1 -> LpositionLampWarning/3  "<VINP_CANMsgValidZONEFR1_flg>"
  LpositionLampWarning/1 -> VINP_LpositionLampWarning_flg/1  "VINP_LpositionLampWarning_flg"
  LpositionLampWarning/2 -> Terminator_17/1
  [BHAL_outputs] -> slr_VHAL_RADBHibeamIndication_flg/1
  slr_VHAL_RADBHibeamIndication_flg/1 -> RADBHibeamIndication/1  "<VHAL_RADBHibeamIndication_flg>"
  True_VHAL_RADBHibeamIndication_flg/1 -> RADBHibeamIndication/2
  [inp_CanValid_bus] -> slr1_18/1
  slr1_18/1 -> RADBHibeamIndication/3  "<VINP_CANMsgValidZONEFR1_flg>"
  RADBHibeamIndication/1 -> VINP_RADBHibeamIndication_flg/1  "VINP_RADBHibeamIndication_flg"
  RADBHibeamIndication/2 -> Terminator_18/1
  [BHAL_outputs] -> slr_VHAL_RADBOperationStatus_flg/1
  slr_VHAL_RADBOperationStatus_flg/1 -> RADBOperationStatus/1  "<VHAL_RADBOperationStatus_flg>"
  True_VHAL_RADBOperationStatus_flg/1 -> RADBOperationStatus/2
  [inp_CanValid_bus] -> slr1_19/1
  slr1_19/1 -> RADBOperationStatus/3  "<VINP_CANMsgValidZONEFR1_flg>"
  RADBOperationStatus/1 -> VINP_RADBOperationStatus_flg/1  "VINP_RADBOperationStatus_flg"
  RADBOperationStatus/2 -> Terminator_19/1
  [BHAL_outputs] -> slr_VHAL_RADBWarning_flg/1
  slr_VHAL_RADBWarning_flg/1 -> RADBWarning/1  "<VHAL_RADBWarning_flg>"
  True_VHAL_RADBWarning_flg/1 -> RADBWarning/2
  [inp_CanValid_bus] -> slr1_20/1
  slr1_20/1 -> RADBWarning/3  "<VINP_CANMsgValidZONEFR1_flg>"
  RADBWarning/1 -> VINP_RADBWarning_flg/1  "VINP_RADBWarning_flg"
  RADBWarning/2 -> Terminator_20/1
  [BHAL_outputs] -> slr_VHAL_RAHBWarning_flg/1
  slr_VHAL_RAHBWarning_flg/1 -> RAHBWarning/1  "<VHAL_RAHBWarning_flg>"
  True_VHAL_RAHBWarning_flg/1 -> RAHBWarning/2
  [inp_CanValid_bus] -> slr1_21/1
  slr1_21/1 -> RAHBWarning/3  "<VINP_CANMsgValidZONEFR1_flg>"
  RAHBWarning/1 -> VINP_RAHBWarning_flg/1  "VINP_RAHBWarning_flg"
  RAHBWarning/2 -> Terminator_21/1
  [BHAL_outputs] -> slr_VHAL_RDRLWarning_flg/1
  slr_VHAL_RDRLWarning_flg/1 -> RDRLWarning/1  "<VHAL_RDRLWarning_flg>"
  True_VHAL_RDRLWarning_flg/1 -> RDRLWarning/2
  [inp_CanValid_bus] -> slr1_22/1
  slr1_22/1 -> RDRLWarning/3  "<VINP_CANMsgValidZONEFR1_flg>"
  RDRLWarning/1 -> VINP_RDRLWarning_flg/1  "VINP_RDRLWarning_flg"
  RDRLWarning/2 -> Terminator_22/1
  [BHAL_outputs] -> slr_VHAL_RLBWarning_flg/1
  slr_VHAL_RLBWarning_flg/1 -> RLBWarning/1  "<VHAL_RLBWarning_flg>"
  True_VHAL_RLBWarning_flg/1 -> RLBWarning/2
  [inp_CanValid_bus] -> slr1_23/1
  slr1_23/1 -> RLBWarning/3  "<VINP_CANMsgValidZONEFR1_flg>"
  RLBWarning/1 -> VINP_RLBWarning_flg/1  "VINP_RLBWarning_flg"
  RLBWarning/2 -> Terminator_23/1
  [BHAL_outputs] -> slr_VHAL_RpositionLampWarning_flg/1
  slr_VHAL_RpositionLampWarning_flg/1 -> RpositionLampWarning/1  "<VHAL_RpositionLampWarning_flg>"
  True_VHAL_RpositionLampWarning_flg/1 -> RpositionLampWarning/2
  [inp_CanValid_bus] -> slr1_24/1
  slr1_24/1 -> RpositionLampWarning/3  "<VINP_CANMsgValidZONEFR1_flg>"
  RpositionLampWarning/1 -> VINP_RpositionLampWarning_flg/1  "VINP_RpositionLampWarning_flg"
  RpositionLampWarning/2 -> Terminator_24/1
  [BHAL_outputs] -> slr_VHAL_TrailerCheck_flg/1
  slr_VHAL_TrailerCheck_flg/1 -> TrailerCheck/1  "<VHAL_TrailerCheck_flg>"
  True_VHAL_TrailerCheck_flg/1 -> TrailerCheck/2
  [inp_CanValid_bus] -> slr1_25/1
  slr1_25/1 -> TrailerCheck/3  "<VINP_CANMsgValidZONEFR1_flg>"
  TrailerCheck/1 -> VINP_TrailerCheck_flg/1  "VINP_TrailerCheck_flg"
  TrailerCheck/2 -> Terminator_25/1
  [BHAL_outputs] -> slr_VHAL_TrailerModeSta_enum/1
  slr_VHAL_TrailerModeSta_enum/1 -> TrailerModeSta/1  "<VHAL_TrailerModeSta_enum>"
  True_VHAL_TrailerModeSta_enum/1 -> TrailerModeSta/2
  [inp_CanValid_bus] -> slr1_26/1
  slr1_26/1 -> TrailerModeSta/3  "<VINP_CANMsgValidZONEFR1_flg>"
  TrailerModeSta/1 -> VINP_TrailerModeSta_enum/1  "VINP_TrailerModeSta_enum"
  TrailerModeSta/2 -> Terminator_26/1
  [BHAL_outputs] -> slr_VHAL_ZFRBCMChargerDoorSWSta_flg/1
  slr_VHAL_ZFRBCMChargerDoorSWSta_flg/1 -> ZFRBCMChargerDoorSWSta/1  "<VHAL_ZFRBCMChargerDoorSWSta_flg>"
  True_VHAL_ZFRBCMChargerDoorSWSta_flg/1 -> ZFRBCMChargerDoorSWSta/2
  [inp_CanValid_bus] -> slr1_27/1
  slr1_27/1 -> ZFRBCMChargerDoorSWSta/3  "<VINP_CANMsgValidZONEFR1_flg>"
  ZFRBCMChargerDoorSWSta/1 -> VINP_ZFRBCMChargerDoorSWSta_flg/1  "VINP_ZFRBCMChargerDoorSWSta_flg"
  ZFRBCMChargerDoorSWSta/2 -> Terminator_27/1
  [BHAL_outputs] -> slr_VHAL_ZFRBCMHRLTurnLPNormalSta_flg/1
  slr_VHAL_ZFRBCMHRLTurnLPNormalSta_flg/1 -> ZFRBCMHRLTurnLPNormalSta/1  "<VHAL_ZFRBCMHRLTurnLPNormalSta_flg>"
  True_VHAL_ZFRBCMHRLTurnLPNormalSta_flg/1 -> ZFRBCMHRLTurnLPNormalSta/2
  [inp_CanValid_bus] -> slr1_28/1
  slr1_28/1 -> ZFRBCMHRLTurnLPNormalSta/3  "<VINP_CANMsgValidZONEFR1_flg>"
  ZFRBCMHRLTurnLPNormalSta/1 -> VINP_ZFRBCMHRLTurnLPNormalSta_flg/1  "VINP_ZFRBCMHRLTurnLPNormalSta_flg"
  ZFRBCMHRLTurnLPNormalSta/2 -> Terminator_28/1
  [BHAL_outputs] -> slr_VHAL_ZFRBCMHRRTurnLPHNormalSta_flg/1
  slr_VHAL_ZFRBCMHRRTurnLPHNormalSta_flg/1 -> ZFRBCMHRRTurnLPHNormalSta/1  "<VHAL_ZFRBCMHRRTurnLPHNormalSta_flg>"
  True_VHAL_ZFRBCMHRRTurnLPHNormalSta_flg/1 -> ZFRBCMHRRTurnLPHNormalSta/2
  [inp_CanValid_bus] -> slr1_29/1
  slr1_29/1 -> ZFRBCMHRRTurnLPHNormalSta/3  "<VINP_CANMsgValidZONEFR1_flg>"
  ZFRBCMHRRTurnLPHNormalSta/1 -> VINP_ZFRBCMHRRTurnLPHNormalSta_flg/1  "VINP_ZFRBCMHRRTurnLPHNormalSta_flg"
  ZFRBCMHRRTurnLPHNormalSta/2 -> Terminator_29/1
  [BHAL_outputs] -> slr_VHAL_ZFRTHCMCLEVentActYSta_pct/1
  slr_VHAL_ZFRTHCMCLEVentActYSta_pct/1 -> ZFRTHCMCLEVentActYSta/1  "<VHAL_ZFRTHCMCLEVentActYSta_pct>"
  True_VHAL_ZFRTHCMCLEVentActYSta_pct/1 -> ZFRTHCMCLEVentActYSta/2
  [inp_CanValid_bus] -> slr1_30/1
  slr1_30/1 -> ZFRTHCMCLEVentActYSta/3  "<VINP_CANMsgValidZONEFR1_flg>"
  ZFRTHCMCLEVentActYSta/1 -> VINP_ZFRTHCMCLEVentActYSta_pct/1  "VINP_ZFRTHCMCLEVentActYSta_pct"
  ZFRTHCMCLEVentActYSta/2 -> Terminator_30/1
  [BHAL_outputs] -> slr_VHAL_ZFRTHCMCREVentActYSta_pct/1
  slr_VHAL_ZFRTHCMCREVentActYSta_pct/1 -> ZFRTHCMCREVentActYSta/1  "<VHAL_ZFRTHCMCREVentActYSta_pct>"
  True_VHAL_ZFRTHCMCREVentActYSta_pct/1 -> ZFRTHCMCREVentActYSta/2
  [inp_CanValid_bus] -> slr1_31/1
  slr1_31/1 -> ZFRTHCMCREVentActYSta/3  "<VINP_CANMsgValidZONEFR1_flg>"
  ZFRTHCMCREVentActYSta/1 -> VINP_ZFRTHCMCREVentActYSta_pct/1  "VINP_ZFRTHCMCREVentActYSta_pct"
  ZFRTHCMCREVentActYSta/2 -> Terminator_31/1
  [BHAL_outputs] -> slr_VHAL_ZFRTHCMDrEVentActYSta_pct/1
  slr_VHAL_ZFRTHCMDrEVentActYSta_pct/1 -> ZFRTHCMDrEVentActYSta/1  "<VHAL_ZFRTHCMDrEVentActYSta_pct>"
  True_VHAL_ZFRTHCMDrEVentActYSta_pct/1 -> ZFRTHCMDrEVentActYSta/2
  [inp_CanValid_bus] -> slr1_32/1
  slr1_32/1 -> ZFRTHCMDrEVentActYSta/3  "<VINP_CANMsgValidZONEFR1_flg>"
  ZFRTHCMDrEVentActYSta/1 -> VINP_ZFRTHCMDrEVentActYSta_pct/1  "VINP_ZFRTHCMDrEVentActYSta_pct"
  ZFRTHCMDrEVentActYSta/2 -> Terminator_32/1
  [BHAL_outputs] -> slr_VHAL_ZFRTHCMPsEVentActYSta_pct/1
  slr_VHAL_ZFRTHCMPsEVentActYSta_pct/1 -> ZFRTHCMPsEVentActYSta/1  "<VHAL_ZFRTHCMPsEVentActYSta_pct>"
  True_VHAL_ZFRTHCMPsEVentActYSta_pct/1 -> ZFRTHCMPsEVentActYSta/2
  [inp_CanValid_bus] -> slr1_33/1
  slr1_33/1 -> ZFRTHCMPsEVentActYSta/3  "<VINP_CANMsgValidZONEFR1_flg>"
  ZFRTHCMPsEVentActYSta/1 -> VINP_ZFRTHCMPsEVentActYSta_pct/1  "VINP_ZFRTHCMPsEVentActYSta_pct"
  ZFRTHCMPsEVentActYSta/2 -> Terminator_33/1
